simulink model "TopLevelSim"  (R2024b)
settings: Solver=FixedStepDiscrete  StartTime=0.0  StopTime=sysParams.FPGAClkPeriod*1e4  RelTol=1e-3
PreLoadFcn:
  | init;
undefined symbols (not defined in the file): bfCoeffs_fxp, chanConfig, const_16APSK, const_64APSK, FXP, iChain, modEnable, modSel, OFDMmodType, SC, SCmodType, sysParams, tuningWord, txData
libraries: hdlsllib x20, commdigbbndpm3 x8, commdigbbndam3 x8, dspmlti4 x8, dsphdlfiltering2 x8, whdlmod x4, dsphdlsigops2 x4
(part 1 of 2)
settings Model: DataTypeOverride=Off  Creator=aless  LastModifiedBy=aless
settings SolverCC: PositivePriorityOrder=on
settings OptimizationCC: BlockReduction=off  ConditionallyExecuteInputs=off  DefaultParameterBehavior=Inlined  InheritOutputTypeSmallerThanSingle=on  EnhancedBackFolding=on  PassReuseOutputArgsAs=Individual arguments  ZeroExternalMemoryAtStartup=off  ZeroInternalMemoryAtStartup=off  MaxStackSize=64  OptimizeBlockOrder=speed  DifferentSizesBufferReuse=on  OptimizationCustomize=off  EfficientTunableParamExpr=on
settings DebuggingCC: AlgebraicLoopMsg=error  SingleTaskRateTransMsg=warning  ParameterTunabilityLossMsg=error  UnconnectedInputMsg=warning  UnconnectedOutputMsg=warning  UnconnectedLineMsg=warning
settings HardwareCC: ProdBitPerPointer=32  ProdBitPerSizeT=32  ProdBitPerPtrDiffT=32  ProdLargestAtomicFloat=None  ProdIntDivRoundTo=Undefined  ProdEndianess=Unspecified  ProdWordSize=32  ProdHWDeviceType=ASIC/FPGA->ASIC/FPGA  TargetBitPerPointer=64  TargetBitPerSizeT=64  TargetBitPerPtrDiffT=64  TargetLongLongMode=on  TargetIntDivRoundTo=Zero  TargetEndianess=LittleEndian  TargetWordSize=64  TargetHWDeviceType=Custom Processor->MATLAB Host Computer  ProdEqTarget=off  HardwareBoardFeatureSet=SoCBlockset
settings ModelReferenceCC: ModelReferenceNumInstancesAllowed=Single
settings RTWCC: Description=Embedded Coder  SystemTargetFile=ert.tlc  HardwareBoard=Xilinx Zynq UltraScale+ RFSoC ZCU208 Evaluation Kit  TLCOptions="-aInlineSetEventsForThisBaseRateFcn=TLC_FALSE -aSuppressMultiTaskScheduler=TLC_FALSE  -aRateBasedStepFcn=0"  TemplateMakefile=ert_default_tmf  Toolchain=Linaro AArch64 Linux v6.3.1
settings CodeAppCC: ForceParamTrailComments=on  IgnoreCustomStorageClasses=off  OperatorAnnotations=on  SimulinkDataObjDesc=on  SFDataObjDesc=on  InsertBlockDesc=on

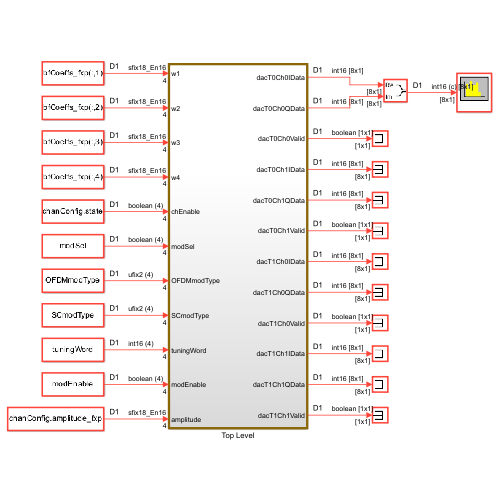
[thumbnail: Simulink's stored preview of the top-level diagram]
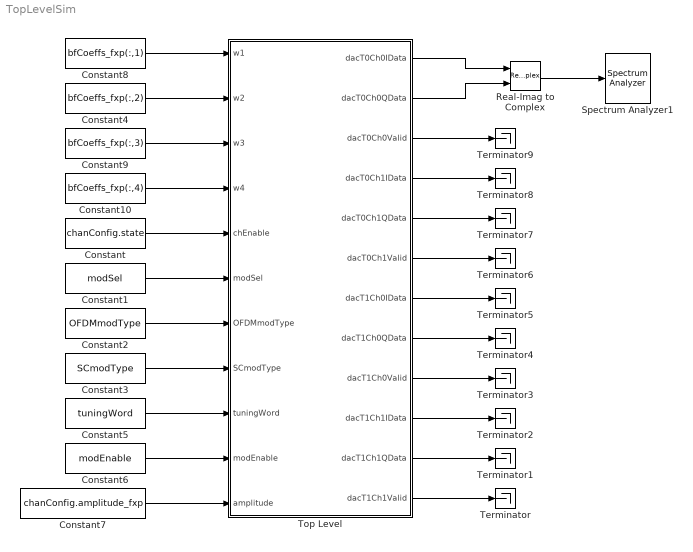
== system TopLevelSim ==
  Constant : Constant  Value=chanConfig.state  OutDataTypeStr=boolean  SampleTime=sysParams.FPGAClkPeriod
  Constant1 : Constant  Value=modSel  OutDataTypeStr=boolean  SampleTime=sysParams.FPGAClkPeriod
  Constant10 : Constant  Value=bfCoeffs_fxp(:,4)  OutDataTypeStr=fixdt(1,FXP.sampWL,FXP.sampFL)  SampleTime=sysParams.FPGAClkPeriod
  Constant2 : Constant  Value=OFDMmodType  OutDataTypeStr=fixdt(0,2,0)  SampleTime=sysParams.FPGAClkPeriod
  Constant3 : Constant  Value=SCmodType  OutDataTypeStr=fixdt(0,2,0)  SampleTime=sysParams.FPGAClkPeriod
  Constant4 : Constant  Value=bfCoeffs_fxp(:,2)  OutDataTypeStr=fixdt(1,FXP.sampWL,FXP.sampFL)  SampleTime=sysParams.FPGAClkPeriod
  Constant5 : Constant  Value=tuningWord  OutDataTypeStr=fixdt(1,FXP.NCOphaseAccWL,0)  SampleTime=sysParams.FPGAClkPeriod
  Constant6 : Constant  Value=modEnable  OutDataTypeStr=boolean  SampleTime=sysParams.FPGAClkPeriod
  Constant7 : Constant  Value=chanConfig.amplitude_fxp  OutDataTypeStr=fixdt(1,FXP.sampWL,FXP.sampFL)  SampleTime=sysParams.FPGAClkPeriod
  Constant8 : Constant  Value=bfCoeffs_fxp(:,1)  OutDataTypeStr=fixdt(1,FXP.sampWL,FXP.sampFL)  SampleTime=sysParams.FPGAClkPeriod
  Constant9 : Constant  Value=bfCoeffs_fxp(:,3)  OutDataTypeStr=fixdt(1,FXP.sampWL,FXP.sampFL)  SampleTime=sysParams.FPGAClkPeriod
  Real-Imag to Complex : RealImagToComplex
  Spectrum Analyzer1 : SpectrumAnalyzer  WindowPosition=[0.000000,36.000000,1536.000000,792.000000,]  ScopeFrameLocation=window  Method=Welch  FrequencyResolutionMethod=Window length  WindowInvariantSamplesPerUpdate=on  WindowLength=4096  FFTLengthSource=Property  FFTLength=8192  Span=1966080000  StartFrequency=-983040000  StopFrequency=983040000  ReferenceLoad=100  YLimits=[-48.29571919,106.76240946]  SelectedToolstripTab=spectrumAnalyzerToolstrip.estimationTab
  Terminator{,1..9} (10 alike) : Terminator
  Top Level : Subsystem  TreatAsAtomicUnit=on
  wires:
  Top Level/1(dacT0Ch0IData) -> Real-Imag to Complex/1
  Top Level/2(dacT0Ch0QData) -> Real-Imag to Complex/2
  Top Level/10(dacT1Ch1IData) -> Terminator2/1
  Top Level/11(dacT1Ch1QData) -> Terminator1/1
  Top Level/12(dacT1Ch1Valid) -> Terminator/1
  Real-Imag to Complex/1 -> Spectrum Analyzer1/1
  Top Level/5(dacT0Ch1QData) -> Terminator7/1
  Top Level/6(dacT0Ch1Valid) -> Terminator6/1
  Top Level/7(dacT1Ch0IData) -> Terminator5/1
  Top Level/8(dacT1Ch0QData) -> Terminator4/1
  Top Level/9(dacT1Ch0Valid) -> Terminator3/1
  Top Level/4(dacT0Ch1IData) -> Terminator8/1
  Top Level/3(dacT0Ch0Valid) -> Terminator9/1
  Constant8/1 -> Top Level/1(w1)
  Constant4/1 -> Top Level/2(w2)
  Constant9/1 -> Top Level/3(w3)
  Constant10/1 -> Top Level/4(w4)
  Constant/1 -> Top Level/5(chEnable)
  Constant1/1 -> Top Level/6(modSel)
  Constant2/1 -> Top Level/7(OFDMmodType)
  Constant3/1 -> Top Level/8(SCmodType)
  Constant5/1 -> Top Level/9(tuningWord)
  Constant6/1 -> Top Level/10(modEnable)
  Constant7/1 -> Top Level/11(amplitude)

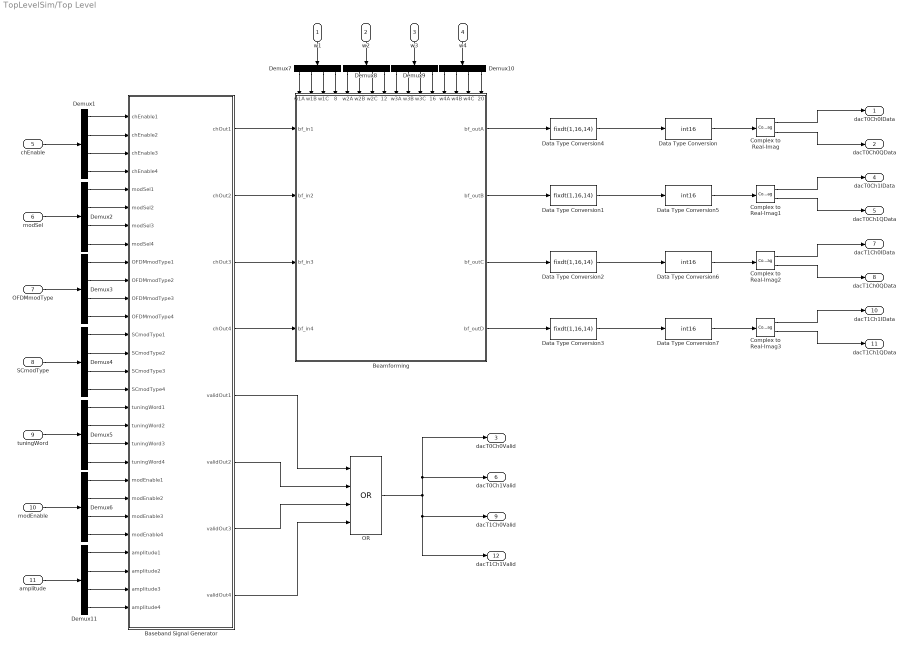
== system TopLevelSim/Top Level ==
  w1 : Inport
  w2 : Inport  Port=2
  w3 : Inport  Port=3
  w4 : Inport  Port=4
  chEnable : Inport  Port=5
  modSel : Inport  Port=6
  OFDMmodType : Inport  Port=7
  SCmodType : Inport  Port=8
  tuningWord : Inport  Port=9
  modEnable : Inport  Port=10
  amplitude : Inport  Port=11
  Baseband Signal Generator : Subsystem
  Beamforming : Subsystem
      settings: PortSchema="{\"entries\":[{\"content\":{\"sides\":[{\"content\":{\"connectorIds\":[\"In1\",\"In2\",\"In3\",\"In4\"]},\"type\":\"ConnectorPlacement.EquallySpacedRectSide\",\"uuid\":\"7b2ca850-5a44-4fe3-a571-bc89de8a8d8a\"},{\"content\":{\"connectorIds\":[\"Out1\",\"Out2\",\"Out3\",\"Out4\"],\"side\":\"RIGHT\"},\"type\":\"ConnectorPlacement.EquallySpacedRectSide\",\"uuid\":\"6a3de6dc-f4ee-4138-b8b6-8ad549f5ffcd\"},{\"content\":{\"connectorIds\":[\"In5\",\"In6\",\"In7\",\"In8\",\"In9\",\"In10\",\"In11\",\"In12\",\"In13\",\"In14\",\"In15\",\"In16\",\"In17\",\"In18\",\"In19\",\"In20\"],\"side\":\"TOP\"},\"type\":\"ConnectorPlacement.EquallySpacedRectSide\",\"uuid\":\"7b227388-a06d-4fee-a646-8c31054e6e12\"}]},\"type\":\"ConnectorPlacement.EquallySpacedConnector\",\"uuid\":\"7849fa84-ba55-4fcd-9e9c-b96e73e847f7\"}],\"packageUris\":[\"http://schema.mathworks.com/mf0/Connector/R2020b\"],\"version\":\"1.0\"}"
  Complex to Real-Imag{,1..3} (4 alike) : ComplexToRealImag
  Data Type Conversion{,5..7} (4 alike) : DataTypeConversion  OutDataTypeStr=int16  ConvertRealWorld=Stored Integer (SI)  SaturateOnIntegerOverflow=off  RndMeth=Floor  LockScale=on
  Data Type Conversion{1..4} (4 alike) : DataTypeConversion  OutDataTypeStr=fixdt(1,16,14)  RndMeth=Nearest  SaturateOnIntegerOverflow=off
  Demux{1..11} (11 alike) : Demux
  OR : Logic  Operator=OR  Inputs=4  AllPortsSameDT=off  OutDataTypeStr=boolean
  dacT0Ch0IData : Outport
  dacT0Ch0QData : Outport  Port=2
  dacT0Ch0Valid : Outport  Port=3
  dacT0Ch1IData : Outport  Port=4
  dacT0Ch1QData : Outport  Port=5
  dacT0Ch1Valid : Outport  Port=6
  dacT1Ch0IData : Outport  Port=7
  dacT1Ch0QData : Outport  Port=8
  dacT1Ch0Valid : Outport  Port=9
  dacT1Ch1IData : Outport  Port=10
  dacT1Ch1QData : Outport  Port=11
  dacT1Ch1Valid : Outport  Port=12
  wires:
  chEnable/1 -> Demux1/1
  SCmodType/1 -> Demux4/1
  OFDMmodType/1 -> Demux3/1
  modSel/1 -> Demux2/1
  modEnable/1 -> Demux6/1
  Data Type Conversion3/1 -> Data Type Conversion7/1
  Complex to Real-Imag3/2 -> dacT1Ch1QData/1
  Baseband Signal Generator/7(validOut3) -> OR/3
  Baseband Signal Generator/3(chOut3) -> Beamforming/3(bf_in3)
  Complex to Real-Imag2/2 -> dacT1Ch0QData/1
  Complex to Real-Imag1/2 -> dacT0Ch1QData/1
  Data Type Conversion2/1 -> Data Type Conversion6/1
  Complex to Real-Imag/1 -> dacT0Ch0IData/1
  Data Type Conversion7/1 -> Complex to Real-Imag3/1
  OR/1 -> dacT0Ch0Valid/1, dacT0Ch1Valid/1, dacT1Ch1Valid/1, dacT1Ch0Valid/1
  Demux7/1 -> Beamforming/5(w1A)
  Beamforming/1(bf_outA) -> Data Type Conversion4/1
  Baseband Signal Generator/6(validOut2) -> OR/2
  Baseband Signal Generator/5(validOut1) -> OR/1
  Complex to Real-Imag1/1 -> dacT0Ch1IData/1
  Complex to Real-Imag2/1 -> dacT1Ch0IData/1
  Baseband Signal Generator/8(validOut4) -> OR/4
  Complex to Real-Imag/2 -> dacT0Ch0QData/1
  Data Type Conversion4/1 -> Data Type Conversion/1
  Baseband Signal Generator/4(chOut4) -> Beamforming/4(bf_in4)
  Baseband Signal Generator/1(chOut1) -> Beamforming/1(bf_in1)
  Beamforming/2(bf_outB) -> Data Type Conversion1/1
  Complex to Real-Imag3/1 -> dacT1Ch1IData/1
  Data Type Conversion6/1 -> Complex to Real-Imag2/1
  Beamforming/4(bf_outD) -> Data Type Conversion3/1
  Data Type Conversion5/1 -> Complex to Real-Imag1/1
  Data Type Conversion1/1 -> Data Type Conversion5/1
  Beamforming/3(bf_outC) -> Data Type Conversion2/1
  Data Type Conversion/1 -> Complex to Real-Imag/1
  Baseband Signal Generator/2(chOut2) -> Beamforming/2(bf_in2)
  Demux7/2 -> Beamforming/6(w1B)
  Demux7/3 -> Beamforming/7(w1C)
  Demux7/4 -> Beamforming/8(w1D)
  Demux8/2 -> Beamforming/10(w2B)
  Demux8/3 -> Beamforming/11(w2C)
  Demux8/4 -> Beamforming/12(w2D)
  Demux8/1 -> Beamforming/9(w2A)
  Demux9/2 -> Beamforming/14(w3B)
  Demux9/3 -> Beamforming/15(w3C)
  Demux9/4 -> Beamforming/16(w3D)
  Demux9/1 -> Beamforming/13(w3A)
  Demux10/2 -> Beamforming/18(w4B)
  Demux10/3 -> Beamforming/19(w4C)
  Demux10/4 -> Beamforming/20(w4D)
  Demux10/1 -> Beamforming/17(w4A)
  w1/1 -> Demux7/1
  w2/1 -> Demux8/1
  w3/1 -> Demux9/1
  w4/1 -> Demux10/1
  tuningWord/1 -> Demux5/1
  amplitude/1 -> Demux11/1
  Demux1/1 -> Baseband Signal Generator/1(chEnable1)
  Demux1/2 -> Baseband Signal Generator/2(chEnable2)
  Demux1/3 -> Baseband Signal Generator/3(chEnable3)
  Demux1/4 -> Baseband Signal Generator/4(chEnable4)
  Demux2/1 -> Baseband Signal Generator/5(modSel1)
  Demux2/2 -> Baseband Signal Generator/6(modSel2)
  Demux2/3 -> Baseband Signal Generator/7(modSel3)
  Demux2/4 -> Baseband Signal Generator/8(modSel4)
  Demux3/1 -> Baseband Signal Generator/9(OFDMmodType1)
  Demux3/2 -> Baseband Signal Generator/10(OFDMmodType2)
  Demux3/3 -> Baseband Signal Generator/11(OFDMmodType3)
  Demux3/4 -> Baseband Signal Generator/12(OFDMmodType4)
  Demux4/1 -> Baseband Signal Generator/13(SCmodType1)
  Demux4/2 -> Baseband Signal Generator/14(SCmodType2)
  Demux4/3 -> Baseband Signal Generator/15(SCmodType3)
  Demux4/4 -> Baseband Signal Generator/16(SCmodType4)
  Demux5/1 -> Baseband Signal Generator/17(tuningWord1)
  Demux5/2 -> Baseband Signal Generator/18(tuningWord2)
  Demux5/3 -> Baseband Signal Generator/19(tuningWord3)
  Demux5/4 -> Baseband Signal Generator/20(tuningWord4)
  Demux6/1 -> Baseband Signal Generator/21(modEnable1)
  Demux6/2 -> Baseband Signal Generator/22(modEnable2)
  Demux6/3 -> Baseband Signal Generator/23(modEnable3)
  Demux6/4 -> Baseband Signal Generator/24(modEnable4)
  Demux11/1 -> Baseband Signal Generator/25(amplitude1)
  Demux11/2 -> Baseband Signal Generator/26(amplitude2)
  Demux11/3 -> Baseband Signal Generator/27(amplitude3)
  Demux11/4 -> Baseband Signal Generator/28(amplitude4)

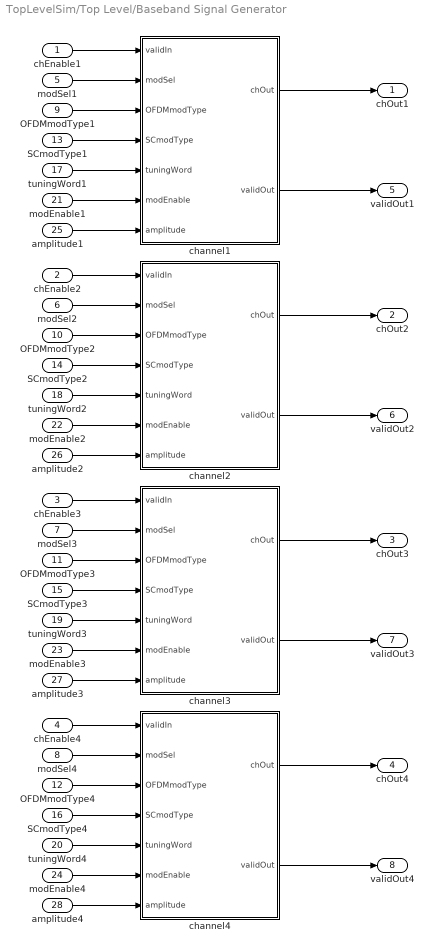
== system TopLevelSim/Top Level/Baseband Signal Generator ==
  chEnable1 : Inport
  chEnable2 : Inport  Port=2
  chEnable3 : Inport  Port=3
  chEnable4 : Inport  Port=4
  modSel1 : Inport  Port=5
  modSel2 : Inport  Port=6
  modSel3 : Inport  Port=7
  modSel4 : Inport  Port=8
  OFDMmodType1 : Inport  Port=9
  OFDMmodType2 : Inport  Port=10
  OFDMmodType3 : Inport  Port=11
  OFDMmodType4 : Inport  Port=12
  SCmodType1 : Inport  Port=13
  SCmodType2 : Inport  Port=14
  SCmodType3 : Inport  Port=15
  SCmodType4 : Inport  Port=16
  tuningWord1 : Inport  Port=17
  tuningWord2 : Inport  Port=18
  tuningWord3 : Inport  Port=19
  tuningWord4 : Inport  Port=20
  modEnable1 : Inport  Port=21
  modEnable2 : Inport  Port=22
  modEnable3 : Inport  Port=23
  modEnable4 : Inport  Port=24
  amplitude1 : Inport  Port=25
  amplitude2 : Inport  Port=26
  amplitude3 : Inport  Port=27
  amplitude4 : Inport  Port=28
  channel1 : Subsystem
  channel2 : Subsystem
  channel3 : Subsystem
  channel4 : Subsystem
  chOut1 : Outport
  chOut2 : Outport  Port=2
  chOut3 : Outport  Port=3
  chOut4 : Outport  Port=4
  validOut1 : Outport  Port=5
  validOut2 : Outport  Port=6
  validOut3 : Outport  Port=7
  validOut4 : Outport  Port=8
  wires:
  tuningWord4/1 -> channel4/5(tuningWord)
  modEnable4/1 -> channel4/6(modEnable)
  modEnable2/1 -> channel2/6(modEnable)
  modEnable1/1 -> channel1/6(modEnable)
  OFDMmodType1/1 -> channel1/3(OFDMmodType)
  modSel1/1 -> channel1/2(modSel)
  tuningWord1/1 -> channel1/5(tuningWord)
  OFDMmodType3/1 -> channel3/3(OFDMmodType)
  channel3/2(validOut) -> validOut3/1
  channel2/1(chOut) -> chOut2/1
  SCmodType1/1 -> channel1/4(SCmodType)
  chEnable2/1 -> channel2/1(validIn)
  channel4/1(chOut) -> chOut4/1
  chEnable1/1 -> channel1/1(validIn)
  channel2/2(validOut) -> validOut2/1
  amplitude1/1 -> channel1/7(amplitude)
  SCmodType3/1 -> channel3/4(SCmodType)
  amplitude4/1 -> channel4/7(amplitude)
  SCmodType4/1 -> channel4/4(SCmodType)
  chEnable4/1 -> channel4/1(validIn)
  modSel4/1 -> channel4/2(modSel)
  OFDMmodType4/1 -> channel4/3(OFDMmodType)
  amplitude2/1 -> channel2/7(amplitude)
  OFDMmodType2/1 -> channel2/3(OFDMmodType)
  SCmodType2/1 -> channel2/4(SCmodType)
  tuningWord3/1 -> channel3/5(tuningWord)
  modSel2/1 -> channel2/2(modSel)
  tuningWord2/1 -> channel2/5(tuningWord)
  modEnable3/1 -> channel3/6(modEnable)
  modSel3/1 -> channel3/2(modSel)
  amplitude3/1 -> channel3/7(amplitude)
  chEnable3/1 -> channel3/1(validIn)
  channel3/1(chOut) -> chOut3/1
  channel4/2(validOut) -> validOut4/1
  channel1/1(chOut) -> chOut1/1
  channel1/2(validOut) -> validOut1/1

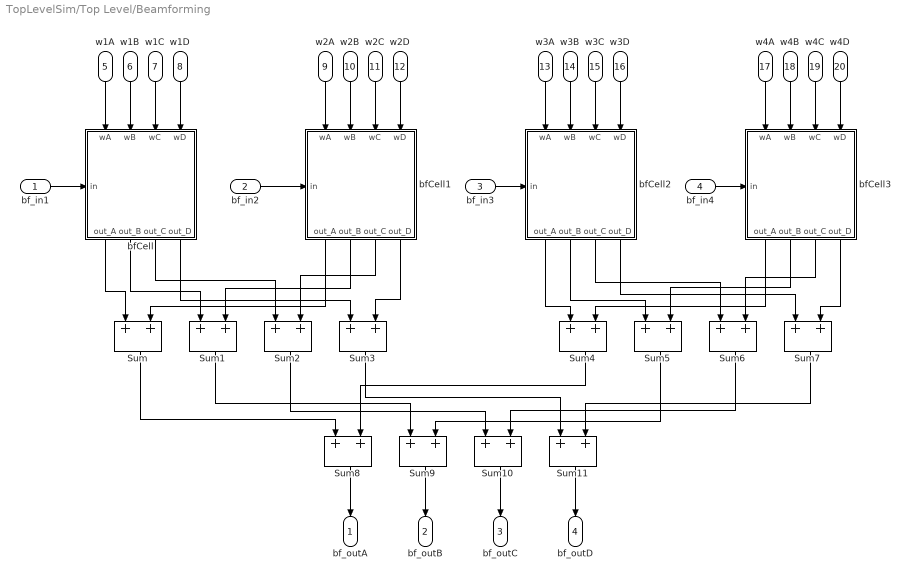
== system TopLevelSim/Top Level/Beamforming ==
  bf_in1 : Inport
  bf_in2 : Inport  Port=2
  bf_in3 : Inport  Port=3
  bf_in4 : Inport  Port=4
  w1A : Inport  Port=5
  w1B : Inport  Port=6
  w1C : Inport  Port=7
  w1D : Inport  Port=8
  w2A : Inport  Port=9
  w2B : Inport  Port=10
  w2C : Inport  Port=11
  w2D : Inport  Port=12
  w3A : Inport  Port=13
  w3B : Inport  Port=14
  w3C : Inport  Port=15
  w3D : Inport  Port=16
  w4A : Inport  Port=17
  w4B : Inport  Port=18
  w4C : Inport  Port=19
  w4D : Inport  Port=20
  Sum{,1..11} (12 alike) : Sum  OutDataTypeStr=Inherit: Same as first input
  bfCell : Subsystem
      settings: PortSchema="{\"entries\":[{\"content\":{\"sides\":[{\"content\":{\"connectorIds\":[\"In1\",\"In2\",\"In3\",\"In4\"]},\"type\":\"ConnectorPlacement.EquallySpacedRectSide\",\"uuid\":\"0c826d6a-73c9-4dba-b1c5-31cfcef02303\"},{\"content\":{\"connectorIds\":[\"Out1\",\"Out2\",\"Out3\",\"Out4\"],\"side\":\"RIGHT\"},\"type\":\"ConnectorPlacement.EquallySpacedRectSide\",\"uuid\":\"e2d5e3de-4ff0-416d-bc8f-a95d356a0a64\"},{\"content\":{\"connectorIds\":[\"In5\"],\"side\":\"TOP\"},\"type\":\"ConnectorPlacement.EquallySpacedRectSide\",\"uuid\":\"bc2266f3-9c70-485a-9b9f-6558f87275cb\"}]},\"type\":\"ConnectorPlacement.EquallySpacedConnector\",\"uuid\":\"4675a578-71f2-44f5-ac97-67035b521010\"}],\"packageUris\":[\"http://schema.mathworks.com/mf0/Connector/R2020b\"],\"version\":\"1.0\"}"
  bfCell1 : Subsystem
      settings: PortSchema="{\"entries\":[{\"content\":{\"sides\":[{\"content\":{\"connectorIds\":[\"In1\",\"In2\",\"In3\",\"In4\"]},\"type\":\"ConnectorPlacement.EquallySpacedRectSide\",\"uuid\":\"0c826d6a-73c9-4dba-b1c5-31cfcef02303\"},{\"content\":{\"connectorIds\":[\"Out1\",\"Out2\",\"Out3\",\"Out4\"],\"side\":\"RIGHT\"},\"type\":\"ConnectorPlacement.EquallySpacedRectSide\",\"uuid\":\"e2d5e3de-4ff0-416d-bc8f-a95d356a0a64\"},{\"content\":{\"connectorIds\":[\"In5\"],\"side\":\"TOP\"},\"type\":\"ConnectorPlacement.EquallySpacedRectSide\",\"uuid\":\"bc2266f3-9c70-485a-9b9f-6558f87275cb\"}]},\"type\":\"ConnectorPlacement.EquallySpacedConnector\",\"uuid\":\"4675a578-71f2-44f5-ac97-67035b521010\"}],\"packageUris\":[\"http://schema.mathworks.com/mf0/Connector/R2020b\"],\"version\":\"1.0\"}"
  bfCell2 : Subsystem
      settings: PortSchema="{\"entries\":[{\"content\":{\"sides\":[{\"content\":{\"connectorIds\":[\"In1\",\"In2\",\"In3\",\"In4\"]},\"type\":\"ConnectorPlacement.EquallySpacedRectSide\",\"uuid\":\"0c826d6a-73c9-4dba-b1c5-31cfcef02303\"},{\"content\":{\"connectorIds\":[\"Out1\",\"Out2\",\"Out3\",\"Out4\"],\"side\":\"RIGHT\"},\"type\":\"ConnectorPlacement.EquallySpacedRectSide\",\"uuid\":\"e2d5e3de-4ff0-416d-bc8f-a95d356a0a64\"},{\"content\":{\"connectorIds\":[\"In5\"],\"side\":\"TOP\"},\"type\":\"ConnectorPlacement.EquallySpacedRectSide\",\"uuid\":\"bc2266f3-9c70-485a-9b9f-6558f87275cb\"}]},\"type\":\"ConnectorPlacement.EquallySpacedConnector\",\"uuid\":\"4675a578-71f2-44f5-ac97-67035b521010\"}],\"packageUris\":[\"http://schema.mathworks.com/mf0/Connector/R2020b\"],\"version\":\"1.0\"}"
  bfCell3 : Subsystem
      settings: PortSchema="{\"entries\":[{\"content\":{\"sides\":[{\"content\":{\"connectorIds\":[\"In1\",\"In2\",\"In3\",\"In4\"]},\"type\":\"ConnectorPlacement.EquallySpacedRectSide\",\"uuid\":\"0c826d6a-73c9-4dba-b1c5-31cfcef02303\"},{\"content\":{\"connectorIds\":[\"Out1\",\"Out2\",\"Out3\",\"Out4\"],\"side\":\"RIGHT\"},\"type\":\"ConnectorPlacement.EquallySpacedRectSide\",\"uuid\":\"e2d5e3de-4ff0-416d-bc8f-a95d356a0a64\"},{\"content\":{\"connectorIds\":[\"In5\"],\"side\":\"TOP\"},\"type\":\"ConnectorPlacement.EquallySpacedRectSide\",\"uuid\":\"bc2266f3-9c70-485a-9b9f-6558f87275cb\"}]},\"type\":\"ConnectorPlacement.EquallySpacedConnector\",\"uuid\":\"4675a578-71f2-44f5-ac97-67035b521010\"}],\"packageUris\":[\"http://schema.mathworks.com/mf0/Connector/R2020b\"],\"version\":\"1.0\"}"
  bf_outA : Outport
  bf_outB : Outport  Port=2
  bf_outC : Outport  Port=3
  bf_outD : Outport  Port=4
  wires:
  Sum8/1 -> bf_outA/1
  Sum9/1 -> bf_outB/1
  Sum10/1 -> bf_outC/1
  Sum11/1 -> bf_outD/1
  w1B/1 -> bfCell/2(wB)
  w1D/1 -> bfCell/4(wD)
  w1A/1 -> bfCell/1(wA)
  w1C/1 -> bfCell/3(wC)
  w2A/1 -> bfCell1/1(wA)
  w2B/1 -> bfCell1/2(wB)
  w2C/1 -> bfCell1/3(wC)
  w2D/1 -> bfCell1/4(wD)
  w3A/1 -> bfCell2/1(wA)
  w3B/1 -> bfCell2/2(wB)
  w3C/1 -> bfCell2/3(wC)
  w3D/1 -> bfCell2/4(wD)
  w4A/1 -> bfCell3/1(wA)
  w4B/1 -> bfCell3/2(wB)
  w4C/1 -> bfCell3/3(wC)
  w4D/1 -> bfCell3/4(wD)
  bf_in1/1 -> bfCell/5(in)
  bf_in2/1 -> bfCell1/5(in)
  bf_in3/1 -> bfCell2/5(in)
  bf_in4/1 -> bfCell3/5(in)
  bfCell/1(out_A) -> Sum/1
  bfCell1/1(out_A) -> Sum/2
  bfCell/2(out_B) -> Sum1/1
  bfCell1/2(out_B) -> Sum1/2
  bfCell/3(out_C) -> Sum2/1
  bfCell1/3(out_C) -> Sum2/2
  bfCell/4(out_D) -> Sum3/1
  bfCell1/4(out_D) -> Sum3/2
  bfCell2/1(out_A) -> Sum4/1
  bfCell3/1(out_A) -> Sum4/2
  bfCell2/2(out_B) -> Sum5/1
  bfCell3/2(out_B) -> Sum5/2
  bfCell2/3(out_C) -> Sum6/1
  bfCell3/3(out_C) -> Sum6/2
  bfCell2/4(out_D) -> Sum7/1
  bfCell3/4(out_D) -> Sum7/2
  Sum/1 -> Sum8/1
  Sum4/1 -> Sum8/2
  Sum1/1 -> Sum9/1
  Sum2/1 -> Sum10/1
  Sum5/1 -> Sum9/2
  Sum6/1 -> Sum10/2
  Sum3/1 -> Sum11/1
  Sum7/1 -> Sum11/2

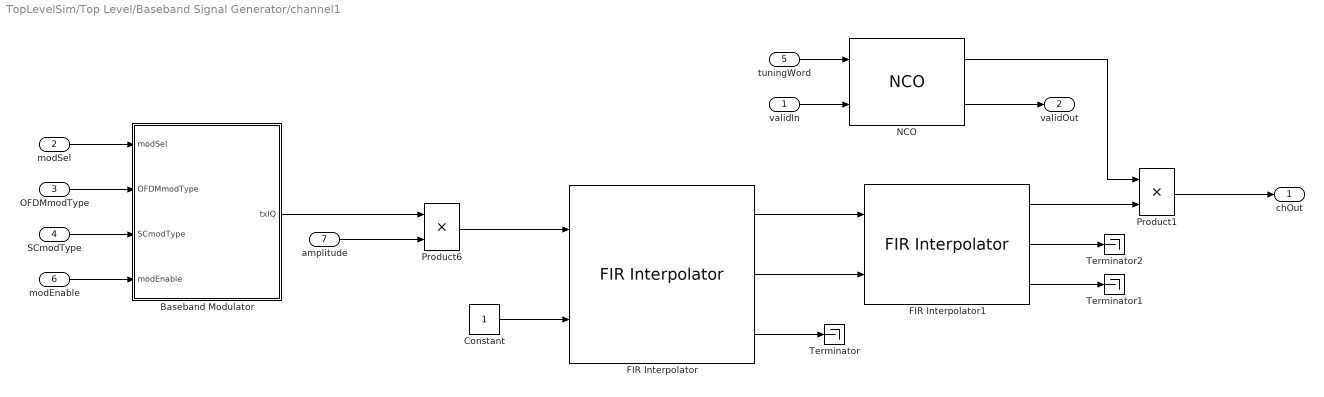
== system TopLevelSim/Top Level/Baseband Signal Generator/channel1 ==
  validIn : Inport
  modSel : Inport  Port=2
  OFDMmodType : Inport  Port=3
  SCmodType : Inport  Port=4
  tuningWord : Inport  Port=5
  modEnable : Inport  Port=6
  amplitude : Inport  Port=7
  Baseband Modulator : Subsystem
  Constant : Constant  OutDataTypeStr=boolean  SampleTime=sysParams.FPGAClkPeriod
  FIR Interpolator : dsphdlfiltering2/FIR Interpolator  Numerator=iChain.firTaps  FilterStructure=Direct form systolic  InterpolationFactor=4  NumCycles=1  OptimizeSymmCoeff=on  SimulateUsing=Code generation  roundingMode=Floor  overflowMode=off  CoefficientsDataTypeStr=fixdt(1,FXP.coeffWL,FXP.coeffFL)  OutputDataTypeStr=fixdt(1,FXP.sampWL,FXP.sampFL)  ResetInputPort=off  HDLGlobalReset=off
  FIR Interpolator1 : dsphdlfiltering2/FIR Interpolator  Numerator=iChain.hbTaps  FilterStructure=Direct form systolic  InterpolationFactor=2  NumCycles=1  OptimizeSymmCoeff=off  SimulateUsing=Code generation  roundingMode=Floor  overflowMode=off  CoefficientsDataTypeStr=fixdt(1,FXP.coeffWL,FXP.coeffFL)  OutputDataTypeStr=fixdt(1,FXP.sampWL,FXP.sampFL)  ResetInputPort=off  HDLGlobalReset=off
  NCO : dsphdlsigops2/NCO  PhaseIncrementSource=Input port  PhaseIncrement=100  PhaseOffsetSource=Property  PhaseOffset=0  DitherSource=None  NumDitherBits=4  SamplesPerFrame=iChain.interpFactor  LUTCompress=on  ResetAction=off  Waveform=Complex exponential  PhasePort=off  SimulateUsing=Code generation  AccumulatorWL=FXP.NCOphaseAccWL  PhaseQuantization=on  NumQuantizerAccumulatorBits=FXP.NCOlutAddressWL  OutputDataType=Binary point scaling  OutputWL=FXP.sampWL  OutputFL=FXP.sampFL
  Product1 : Product  OutDataTypeStr=fixdt(1,FXP.sampWL,FXP.sampFL)
  Product6 : Product  OutDataTypeStr=fixdt(1,FXP.sampWL,FXP.sampFL)
  Terminator : Terminator
  Terminator1 : Terminator
  Terminator2 : Terminator
  chOut : Outport
  validOut : Outport  Port=2
  wires:
  FIR Interpolator1/3 -> Terminator1/1
  SCmodType/1 -> Baseband Modulator/3(SCmodType)
  tuningWord/1 -> NCO/1
  modSel/1 -> Baseband Modulator/1(modSel)
  OFDMmodType/1 -> Baseband Modulator/2(OFDMmodType)
  modEnable/1 -> Baseband Modulator/4(modEnable)
  FIR Interpolator/3 -> Terminator/1
  Baseband Modulator/1(txIQ) -> Product6/1
  validIn/1 -> NCO/2
  amplitude/1 -> Product6/2
  Product6/1 -> FIR Interpolator/1
  Product1/1 -> chOut/1
  FIR Interpolator/1 -> FIR Interpolator1/1
  FIR Interpolator/2 -> FIR Interpolator1/2
  NCO/2 -> validOut/1
  Constant/1 -> FIR Interpolator/2
  FIR Interpolator1/2 -> Terminator2/1
  FIR Interpolator1/1 -> Product1/2
  NCO/1 -> Product1/1

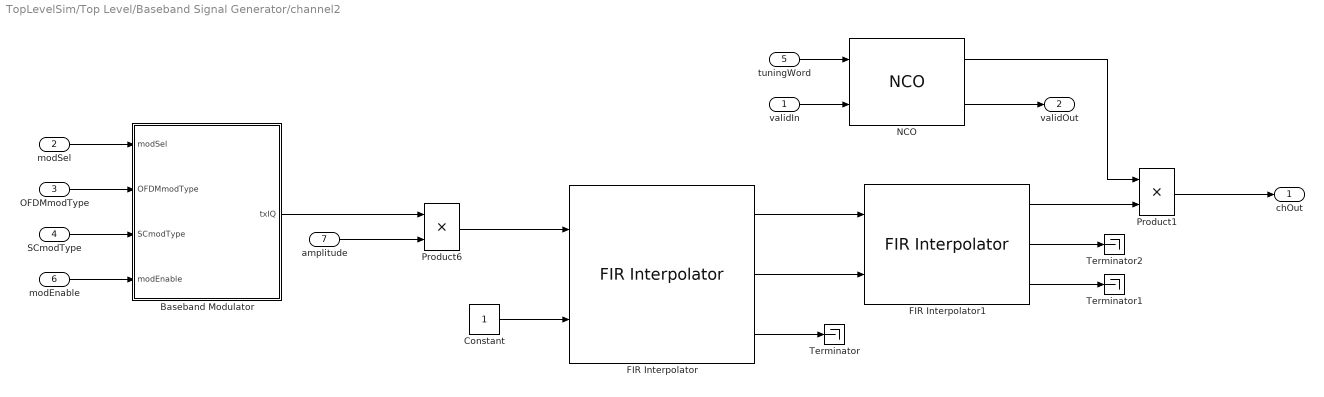
== system TopLevelSim/Top Level/Baseband Signal Generator/channel2 ==
  validIn : Inport
  modSel : Inport  Port=2
  OFDMmodType : Inport  Port=3
  SCmodType : Inport  Port=4
  tuningWord : Inport  Port=5
  modEnable : Inport  Port=6
  amplitude : Inport  Port=7
  Baseband Modulator : Subsystem
  Constant : Constant  OutDataTypeStr=boolean  SampleTime=sysParams.FPGAClkPeriod
  FIR Interpolator : dsphdlfiltering2/FIR Interpolator  Numerator=iChain.firTaps  FilterStructure=Direct form systolic  InterpolationFactor=4  NumCycles=1  OptimizeSymmCoeff=on  SimulateUsing=Code generation  roundingMode=Floor  overflowMode=off  CoefficientsDataTypeStr=fixdt(1,FXP.coeffWL,FXP.coeffFL)  OutputDataTypeStr=fixdt(1,FXP.sampWL,FXP.sampFL)  ResetInputPort=off  HDLGlobalReset=off
  FIR Interpolator1 : dsphdlfiltering2/FIR Interpolator  Numerator=iChain.hbTaps  FilterStructure=Direct form systolic  InterpolationFactor=2  NumCycles=1  OptimizeSymmCoeff=off  SimulateUsing=Code generation  roundingMode=Floor  overflowMode=off  CoefficientsDataTypeStr=fixdt(1,FXP.coeffWL,FXP.coeffFL)  OutputDataTypeStr=fixdt(1,FXP.sampWL,FXP.sampFL)  ResetInputPort=off  HDLGlobalReset=off
  NCO : dsphdlsigops2/NCO  PhaseIncrementSource=Input port  PhaseIncrement=100  PhaseOffsetSource=Property  PhaseOffset=0  DitherSource=None  NumDitherBits=4  SamplesPerFrame=iChain.interpFactor  LUTCompress=on  ResetAction=off  Waveform=Complex exponential  PhasePort=off  SimulateUsing=Code generation  AccumulatorWL=FXP.NCOphaseAccWL  PhaseQuantization=on  NumQuantizerAccumulatorBits=FXP.NCOlutAddressWL  OutputDataType=Binary point scaling  OutputWL=FXP.sampWL  OutputFL=FXP.sampFL
  Product1 : Product  OutDataTypeStr=fixdt(1,FXP.sampWL,FXP.sampFL)
  Product6 : Product  OutDataTypeStr=fixdt(1,FXP.sampWL,FXP.sampFL)
  Terminator : Terminator
  Terminator1 : Terminator
  Terminator2 : Terminator
  chOut : Outport
  validOut : Outport  Port=2
  wires:
  NCO/1 -> Product1/1
  FIR Interpolator1/1 -> Product1/2
  FIR Interpolator1/2 -> Terminator2/1
  Constant/1 -> FIR Interpolator/2
  NCO/2 -> validOut/1
  FIR Interpolator/2 -> FIR Interpolator1/2
  FIR Interpolator/1 -> FIR Interpolator1/1
  Product1/1 -> chOut/1
  Product6/1 -> FIR Interpolator/1
  amplitude/1 -> Product6/2
  validIn/1 -> NCO/2
  Baseband Modulator/1(txIQ) -> Product6/1
  FIR Interpolator/3 -> Terminator/1
  modEnable/1 -> Baseband Modulator/4(modEnable)
  OFDMmodType/1 -> Baseband Modulator/2(OFDMmodType)
  modSel/1 -> Baseband Modulator/1(modSel)
  tuningWord/1 -> NCO/1
  SCmodType/1 -> Baseband Modulator/3(SCmodType)
  FIR Interpolator1/3 -> Terminator1/1

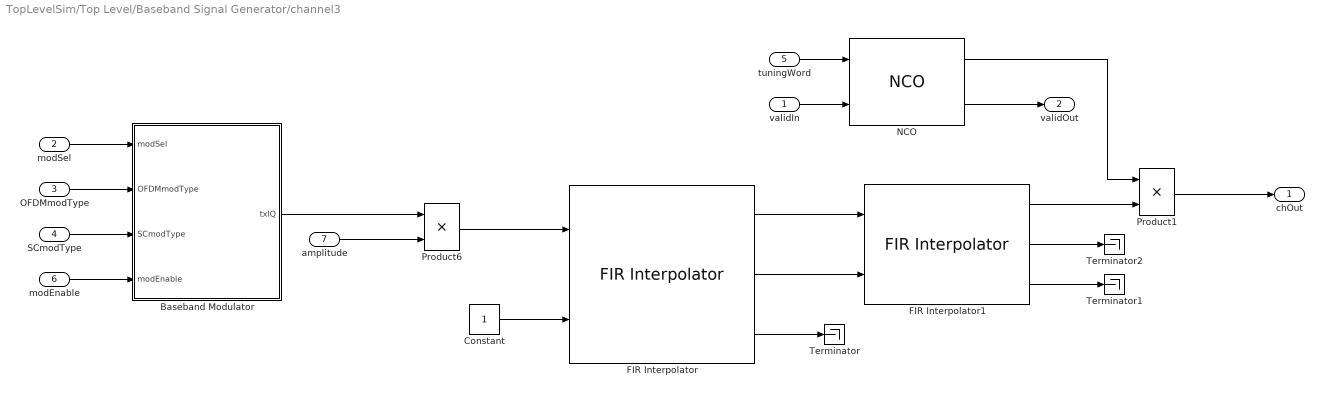
== system TopLevelSim/Top Level/Baseband Signal Generator/channel3 ==
  validIn : Inport
  modSel : Inport  Port=2
  OFDMmodType : Inport  Port=3
  SCmodType : Inport  Port=4
  tuningWord : Inport  Port=5
  modEnable : Inport  Port=6
  amplitude : Inport  Port=7
  Baseband Modulator : Subsystem
  Constant : Constant  OutDataTypeStr=boolean  SampleTime=sysParams.FPGAClkPeriod
  FIR Interpolator : dsphdlfiltering2/FIR Interpolator  Numerator=iChain.firTaps  FilterStructure=Direct form systolic  InterpolationFactor=4  NumCycles=1  OptimizeSymmCoeff=on  SimulateUsing=Code generation  roundingMode=Floor  overflowMode=off  CoefficientsDataTypeStr=fixdt(1,FXP.coeffWL,FXP.coeffFL)  OutputDataTypeStr=fixdt(1,FXP.sampWL,FXP.sampFL)  ResetInputPort=off  HDLGlobalReset=off
  FIR Interpolator1 : dsphdlfiltering2/FIR Interpolator  Numerator=iChain.hbTaps  FilterStructure=Direct form systolic  InterpolationFactor=2  NumCycles=1  OptimizeSymmCoeff=off  SimulateUsing=Code generation  roundingMode=Floor  overflowMode=off  CoefficientsDataTypeStr=fixdt(1,FXP.coeffWL,FXP.coeffFL)  OutputDataTypeStr=fixdt(1,FXP.sampWL,FXP.sampFL)  ResetInputPort=off  HDLGlobalReset=off
  NCO : dsphdlsigops2/NCO  PhaseIncrementSource=Input port  PhaseIncrement=100  PhaseOffsetSource=Property  PhaseOffset=0  DitherSource=None  NumDitherBits=4  SamplesPerFrame=iChain.interpFactor  LUTCompress=on  ResetAction=off  Waveform=Complex exponential  PhasePort=off  SimulateUsing=Code generation  AccumulatorWL=FXP.NCOphaseAccWL  PhaseQuantization=on  NumQuantizerAccumulatorBits=FXP.NCOlutAddressWL  OutputDataType=Binary point scaling  OutputWL=FXP.sampWL  OutputFL=FXP.sampFL
  Product1 : Product  OutDataTypeStr=fixdt(1,FXP.sampWL,FXP.sampFL)
  Product6 : Product  OutDataTypeStr=fixdt(1,FXP.sampWL,FXP.sampFL)
  Terminator : Terminator
  Terminator1 : Terminator
  Terminator2 : Terminator
  chOut : Outport
  validOut : Outport  Port=2
  wires:
  FIR Interpolator1/3 -> Terminator1/1
  SCmodType/1 -> Baseband Modulator/3(SCmodType)
  tuningWord/1 -> NCO/1
  modSel/1 -> Baseband Modulator/1(modSel)
  OFDMmodType/1 -> Baseband Modulator/2(OFDMmodType)
  modEnable/1 -> Baseband Modulator/4(modEnable)
  FIR Interpolator/3 -> Terminator/1
  Baseband Modulator/1(txIQ) -> Product6/1
  validIn/1 -> NCO/2
  amplitude/1 -> Product6/2
  Product6/1 -> FIR Interpolator/1
  Product1/1 -> chOut/1
  FIR Interpolator/1 -> FIR Interpolator1/1
  FIR Interpolator/2 -> FIR Interpolator1/2
  NCO/2 -> validOut/1
  Constant/1 -> FIR Interpolator/2
  FIR Interpolator1/2 -> Terminator2/1
  FIR Interpolator1/1 -> Product1/2
  NCO/1 -> Product1/1

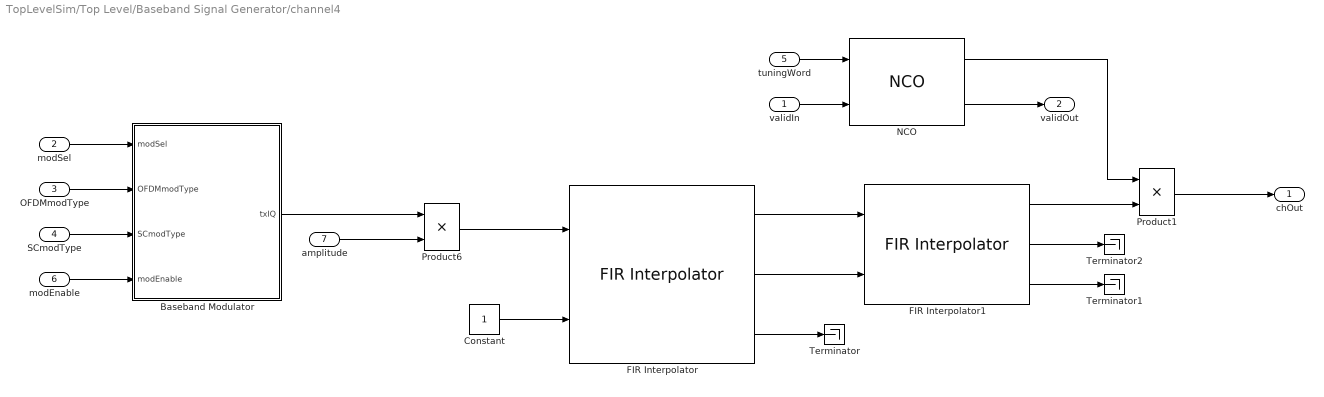
== system TopLevelSim/Top Level/Baseband Signal Generator/channel4 ==
  validIn : Inport
  modSel : Inport  Port=2
  OFDMmodType : Inport  Port=3
  SCmodType : Inport  Port=4
  tuningWord : Inport  Port=5
  modEnable : Inport  Port=6
  amplitude : Inport  Port=7
  Baseband Modulator : Subsystem
  Constant : Constant  OutDataTypeStr=boolean  SampleTime=sysParams.FPGAClkPeriod
  FIR Interpolator : dsphdlfiltering2/FIR Interpolator  Numerator=iChain.firTaps  FilterStructure=Direct form systolic  InterpolationFactor=4  NumCycles=1  OptimizeSymmCoeff=on  SimulateUsing=Code generation  roundingMode=Floor  overflowMode=off  CoefficientsDataTypeStr=fixdt(1,FXP.coeffWL,FXP.coeffFL)  OutputDataTypeStr=fixdt(1,FXP.sampWL,FXP.sampFL)  ResetInputPort=off  HDLGlobalReset=off
  FIR Interpolator1 : dsphdlfiltering2/FIR Interpolator  Numerator=iChain.hbTaps  FilterStructure=Direct form systolic  InterpolationFactor=2  NumCycles=1  OptimizeSymmCoeff=off  SimulateUsing=Code generation  roundingMode=Floor  overflowMode=off  CoefficientsDataTypeStr=fixdt(1,FXP.coeffWL,FXP.coeffFL)  OutputDataTypeStr=fixdt(1,FXP.sampWL,FXP.sampFL)  ResetInputPort=off  HDLGlobalReset=off
  NCO : dsphdlsigops2/NCO  PhaseIncrementSource=Input port  PhaseIncrement=100  PhaseOffsetSource=Property  PhaseOffset=0  DitherSource=None  NumDitherBits=4  SamplesPerFrame=iChain.interpFactor  LUTCompress=on  ResetAction=off  Waveform=Complex exponential  PhasePort=off  SimulateUsing=Code generation  AccumulatorWL=FXP.NCOphaseAccWL  PhaseQuantization=on  NumQuantizerAccumulatorBits=FXP.NCOlutAddressWL  OutputDataType=Binary point scaling  OutputWL=FXP.sampWL  OutputFL=FXP.sampFL
  Product1 : Product  OutDataTypeStr=fixdt(1,FXP.sampWL,FXP.sampFL)
  Product6 : Product  OutDataTypeStr=fixdt(1,FXP.sampWL,FXP.sampFL)
  Terminator : Terminator
  Terminator1 : Terminator
  Terminator2 : Terminator
  chOut : Outport
  validOut : Outport  Port=2
  wires:
  NCO/1 -> Product1/1
  FIR Interpolator1/1 -> Product1/2
  FIR Interpolator1/2 -> Terminator2/1
  Constant/1 -> FIR Interpolator/2
  NCO/2 -> validOut/1
  FIR Interpolator/2 -> FIR Interpolator1/2
  FIR Interpolator/1 -> FIR Interpolator1/1
  Product1/1 -> chOut/1
  Product6/1 -> FIR Interpolator/1
  amplitude/1 -> Product6/2
  validIn/1 -> NCO/2
  Baseband Modulator/1(txIQ) -> Product6/1
  FIR Interpolator/3 -> Terminator/1
  modEnable/1 -> Baseband Modulator/4(modEnable)
  OFDMmodType/1 -> Baseband Modulator/2(OFDMmodType)
  modSel/1 -> Baseband Modulator/1(modSel)
  tuningWord/1 -> NCO/1
  SCmodType/1 -> Baseband Modulator/3(SCmodType)
  FIR Interpolator1/3 -> Terminator1/1

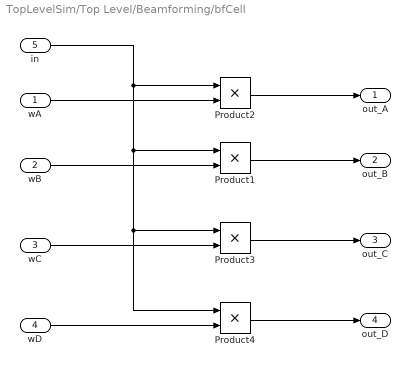
== system TopLevelSim/Top Level/Beamforming/bfCell ==
  wA : Inport
  wB : Inport  Port=2
  wC : Inport  Port=3
  wD : Inport  Port=4
  in : Inport  Port=5
  Product{1..4} (4 alike) : Product  OutDataTypeStr=fixdt(1,FXP.sampWL,FXP.sampFL)
  out_A : Outport
  out_B : Outport  Port=2
  out_C : Outport  Port=3
  out_D : Outport  Port=4
  wires:
  wB/1 -> Product1/2
  in/1 -> Product2/1, Product1/1, Product4/1, Product3/1
  wC/1 -> Product3/2
  wD/1 -> Product4/2
  Product3/1 -> out_C/1
  Product1/1 -> out_B/1
  Product4/1 -> out_D/1
  Product2/1 -> out_A/1
  wA/1 -> Product2/2

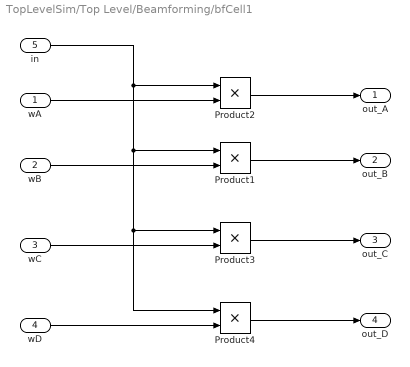
== system TopLevelSim/Top Level/Beamforming/bfCell1 ==
  wA : Inport
  wB : Inport  Port=2
  wC : Inport  Port=3
  wD : Inport  Port=4
  in : Inport  Port=5
  Product{1..4} (4 alike) : Product  OutDataTypeStr=fixdt(1,FXP.sampWL,FXP.sampFL)
  out_A : Outport
  out_B : Outport  Port=2
  out_C : Outport  Port=3
  out_D : Outport  Port=4
  wires:
  wA/1 -> Product2/2
  Product2/1 -> out_A/1
  Product4/1 -> out_D/1
  Product1/1 -> out_B/1
  Product3/1 -> out_C/1
  wD/1 -> Product4/2
  wC/1 -> Product3/2
  in/1 -> Product3/1, Product4/1, Product1/1, Product2/1
  wB/1 -> Product1/2

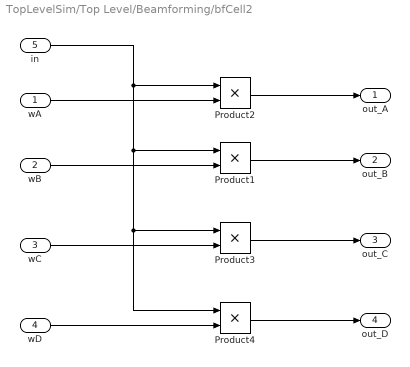
== system TopLevelSim/Top Level/Beamforming/bfCell2 ==
  wA : Inport
  wB : Inport  Port=2
  wC : Inport  Port=3
  wD : Inport  Port=4
  in : Inport  Port=5
  Product{1..4} (4 alike) : Product  OutDataTypeStr=fixdt(1,FXP.sampWL,FXP.sampFL)
  out_A : Outport
  out_B : Outport  Port=2
  out_C : Outport  Port=3
  out_D : Outport  Port=4
  wires:
  wB/1 -> Product1/2
  in/1 -> Product2/1, Product1/1, Product4/1, Product3/1
  wC/1 -> Product3/2
  wD/1 -> Product4/2
  Product3/1 -> out_C/1
  Product1/1 -> out_B/1
  Product4/1 -> out_D/1
  Product2/1 -> out_A/1
  wA/1 -> Product2/2

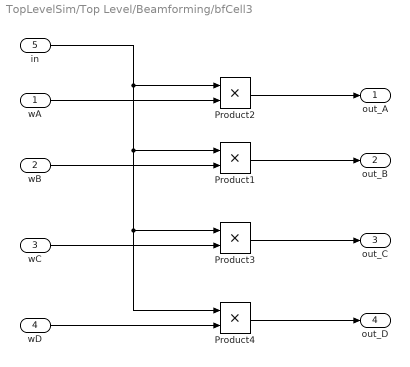
== system TopLevelSim/Top Level/Beamforming/bfCell3 ==
  wA : Inport
  wB : Inport  Port=2
  wC : Inport  Port=3
  wD : Inport  Port=4
  in : Inport  Port=5
  Product{1..4} (4 alike) : Product  OutDataTypeStr=fixdt(1,FXP.sampWL,FXP.sampFL)
  out_A : Outport
  out_B : Outport  Port=2
  out_C : Outport  Port=3
  out_D : Outport  Port=4
  wires:
  wA/1 -> Product2/2
  Product2/1 -> out_A/1
  Product4/1 -> out_D/1
  Product1/1 -> out_B/1
  Product3/1 -> out_C/1
  wD/1 -> Product4/2
  wC/1 -> Product3/2
  in/1 -> Product3/1, Product4/1, Product1/1, Product2/1
  wB/1 -> Product1/2

== system TopLevelSim/Top Level/Baseband Signal Generator/channel1/Baseband Modulator ==
  modSel : Inport
  OFDMmodType : Inport  Port=2
  SCmodType : Inport  Port=3
  modEnable : Inport  Port=4
  Constant2 : Constant  Value=complex(1,0)  OutDataTypeStr=fixdt(1,FXP.sampWL,FXP.sampFL)  SampleTime=sysParams.FPGAClkPeriod
  Counter Free-Running : hdlsllib/Sources/Counter Free-Running  NumBits=lutAddrWidth  tsamp=sysParams.FPGAClkPeriod
  Direct Lookup Table (n-D) : LookupNDDirect  NumberOfTableDimensions=1  Table=txData(:,1)  DiagnosticForOutOfRangeInput=Error
  OFDM Modulator : Subsystem
  SC Modulator : Subsystem
  Switch : Switch  Criteria=u2 > Threshold  OutDataTypeStr=fixdt(1,FXP.sampWL,FXP.sampFL)  SaturateOnIntegerOverflow=off  InputSameDT=off
  Switch1 : Switch  Criteria=u2 > Threshold  OutDataTypeStr=fixdt(1,FXP.sampWL,FXP.sampFL)  SaturateOnIntegerOverflow=off  InputSameDT=off
  txIQ : Outport
  wires:
  OFDMmodType/1 -> OFDM Modulator/2(OFDMmodType)
  Counter Free-Running/1 -> Direct Lookup Table (n-D)/1
  OFDM Modulator/1(txIQ) -> Switch1/3
  Direct Lookup Table (n-D)/1 -> SC Modulator/2(txBits), OFDM Modulator/1(txBits)
  SC Modulator/1(txIQ) -> Switch1/1
  SCmodType/1 -> SC Modulator/1(SCmodType)
  modSel/1 -> Switch1/2
  modEnable/1 -> Switch/2
  Switch1/1 -> Switch/1
  Switch/1 -> txIQ/1
  Constant2/1 -> Switch/3

== system TopLevelSim/Top Level/Baseband Signal Generator/channel2/Baseband Modulator ==
  modSel : Inport
  OFDMmodType : Inport  Port=2
  SCmodType : Inport  Port=3
  modEnable : Inport  Port=4
  Constant2 : Constant  Value=complex(1,0)  OutDataTypeStr=fixdt(1,FXP.sampWL,FXP.sampFL)  SampleTime=sysParams.FPGAClkPeriod
  Counter Free-Running : hdlsllib/Sources/Counter Free-Running  NumBits=lutAddrWidth  tsamp=sysParams.FPGAClkPeriod
  Direct Lookup Table (n-D) : LookupNDDirect  NumberOfTableDimensions=1  Table=txData(:,2)  DiagnosticForOutOfRangeInput=Error
  OFDM Modulator : Subsystem
  SC Modulator : Subsystem
  Switch : Switch  Criteria=u2 > Threshold  OutDataTypeStr=fixdt(1,FXP.sampWL,FXP.sampFL)  SaturateOnIntegerOverflow=off  InputSameDT=off
  Switch1 : Switch  Criteria=u2 > Threshold  OutDataTypeStr=fixdt(1,FXP.sampWL,FXP.sampFL)  SaturateOnIntegerOverflow=off  InputSameDT=off
  txIQ : Outport
  wires:
  Constant2/1 -> Switch/3
  Switch/1 -> txIQ/1
  Switch1/1 -> Switch/1
  modEnable/1 -> Switch/2
  modSel/1 -> Switch1/2
  SCmodType/1 -> SC Modulator/1(SCmodType)
  SC Modulator/1(txIQ) -> Switch1/1
  Direct Lookup Table (n-D)/1 -> OFDM Modulator/1(txBits), SC Modulator/2(txBits)
  OFDM Modulator/1(txIQ) -> Switch1/3
  Counter Free-Running/1 -> Direct Lookup Table (n-D)/1
  OFDMmodType/1 -> OFDM Modulator/2(OFDMmodType)

== system TopLevelSim/Top Level/Baseband Signal Generator/channel3/Baseband Modulator ==
  modSel : Inport
  OFDMmodType : Inport  Port=2
  SCmodType : Inport  Port=3
  modEnable : Inport  Port=4
  Constant2 : Constant  Value=complex(1,0)  OutDataTypeStr=fixdt(1,FXP.sampWL,FXP.sampFL)  SampleTime=sysParams.FPGAClkPeriod
  Counter Free-Running : hdlsllib/Sources/Counter Free-Running  NumBits=lutAddrWidth  tsamp=sysParams.FPGAClkPeriod
  Direct Lookup Table (n-D) : LookupNDDirect  NumberOfTableDimensions=1  Table=txData(:,3)  DiagnosticForOutOfRangeInput=Error
  OFDM Modulator : Subsystem
  SC Modulator : Subsystem
  Switch : Switch  Criteria=u2 > Threshold  OutDataTypeStr=fixdt(1,FXP.sampWL,FXP.sampFL)  SaturateOnIntegerOverflow=off  InputSameDT=off
  Switch1 : Switch  Criteria=u2 > Threshold  OutDataTypeStr=fixdt(1,FXP.sampWL,FXP.sampFL)  SaturateOnIntegerOverflow=off  InputSameDT=off
  txIQ : Outport
  wires:
  OFDMmodType/1 -> OFDM Modulator/2(OFDMmodType)
  Counter Free-Running/1 -> Direct Lookup Table (n-D)/1
  OFDM Modulator/1(txIQ) -> Switch1/3
  Direct Lookup Table (n-D)/1 -> SC Modulator/2(txBits), OFDM Modulator/1(txBits)
  SC Modulator/1(txIQ) -> Switch1/1
  SCmodType/1 -> SC Modulator/1(SCmodType)
  modSel/1 -> Switch1/2
  modEnable/1 -> Switch/2
  Switch1/1 -> Switch/1
  Switch/1 -> txIQ/1
  Constant2/1 -> Switch/3

== system TopLevelSim/Top Level/Baseband Signal Generator/channel4/Baseband Modulator ==
  modSel : Inport
  OFDMmodType : Inport  Port=2
  SCmodType : Inport  Port=3
  modEnable : Inport  Port=4
  Constant2 : Constant  Value=complex(1,0)  OutDataTypeStr=fixdt(1,FXP.sampWL,FXP.sampFL)  SampleTime=sysParams.FPGAClkPeriod
  Counter Free-Running : hdlsllib/Sources/Counter Free-Running  NumBits=lutAddrWidth  tsamp=sysParams.FPGAClkPeriod
  Direct Lookup Table (n-D) : LookupNDDirect  NumberOfTableDimensions=1  Table=txData(:,4)  DiagnosticForOutOfRangeInput=Error
  OFDM Modulator : Subsystem
  SC Modulator : Subsystem
  Switch : Switch  Criteria=u2 > Threshold  OutDataTypeStr=fixdt(1,FXP.sampWL,FXP.sampFL)  SaturateOnIntegerOverflow=off  InputSameDT=off
  Switch1 : Switch  Criteria=u2 > Threshold  OutDataTypeStr=fixdt(1,FXP.sampWL,FXP.sampFL)  SaturateOnIntegerOverflow=off  InputSameDT=off
  txIQ : Outport
  wires:
  Constant2/1 -> Switch/3
  Switch/1 -> txIQ/1
  Switch1/1 -> Switch/1
  modEnable/1 -> Switch/2
  modSel/1 -> Switch1/2
  SCmodType/1 -> SC Modulator/1(SCmodType)
  SC Modulator/1(txIQ) -> Switch1/1
  Direct Lookup Table (n-D)/1 -> OFDM Modulator/1(txBits), SC Modulator/2(txBits)
  OFDM Modulator/1(txIQ) -> Switch1/3
  Counter Free-Running/1 -> Direct Lookup Table (n-D)/1
  OFDMmodType/1 -> OFDM Modulator/2(OFDMmodType)

== system TopLevelSim/Top Level/Baseband Signal Generator/channel1/Baseband Modulator/OFDM Modulator ==
  txBits : Inport
  OFDMmodType : Inport  Port=2
  Constant : Constant  OutDataTypeStr=boolean  SampleTime=sysParams.FPGAClkPeriod
  OFDM Modulator : whdlmod/OFDM Modulator  OFDMParametersSource=Property  FFTLength=OFDM.ifftSize  MaxFFTLength=64  CPLength=OFDM.CpLength  numLgSc=OFDM.numLgSc  numRgSc=OFDM.numRgSc  InsertDCNull=off  Windowing=on  WindowLength=OFDM.WindowLength  MaxWindowLength=8  ResetInputPort=off  Normalize=on  RoundingMethod=Floor  SimulateUsing=Code generation
  Terminator : Terminator
  Terminator1 : Terminator
  mapper : Subsystem
  txIQ : Outport
  wires:
  txBits/1 -> mapper/1(txBits)
  OFDMmodType/1 -> mapper/2(OFDMmodType)
  OFDM Modulator/1 -> txIQ/1
  OFDM Modulator/2 -> Terminator1/1
  mapper/1(tx_IQ) -> OFDM Modulator/1
  OFDM Modulator/3 -> Terminator/1
  Constant/1 -> OFDM Modulator/2

== system TopLevelSim/Top Level/Baseband Signal Generator/channel1/Baseband Modulator/SC Modulator ==
  SCmodType : Inport
  txBits : Inport  Port=2
  FIR Interpolation : dspmlti4/FIR Interpolation  FilterSource=Dialog parameters  PrivateCoeffs=0  h=SC.firTaps  L=SC.firInterpFactor  FilterObject=FINTERP  framing=Allow multirate processing  outputBufInitCond=0  roundingMode=Floor  overflowMode=off  firstCoeffMode=Binary point scaling  firstCoeffWordLength=FXP.coeffWL  firstCoeffFracLength=FXP.coeffFL  firstCoeffDataTypeStr=fixdt(1,FXP.coeffWL,FXP.coeffFL)  firstCoeffMin=[]  firstCoeffMax=[]  firstCoeffLastDataTypeStr=fixdt(1,FXP.coeffWL,FXP.coeffFL)  outputMode=Binary point scaling  outputWordLength=FXP.sampWL  outputFracLength=FXP.sampFL  outputDataTypeStr=fixdt(1,FXP.sampWL,FXP.sampFL)  outputMin=[]  outputMax=[]  outputLastDataTypeStr=fixdt(1,FXP.sampWL,FXP.sampFL)
  Rate Transition : RateTransition  OutPortSampleTimeMultiple=40  OutPortSampleTime=1/SC.symRate
  Root-Raised Cosine : dspmlti4/FIR Interpolation  FilterSource=Dialog parameters  PrivateCoeffs=0  h=SC.RRC.taps  L=SC.RRC.sampPerSym  FilterObject=FINTERP  framing=Allow multirate processing  outputBufInitCond=0  roundingMode=Floor  overflowMode=off  firstCoeffMode=Binary point scaling  firstCoeffWordLength=FXP.coeffWL  firstCoeffFracLength=FXP.coeffFL  firstCoeffDataTypeStr=fixdt(1,FXP.coeffWL,FXP.coeffFL)  firstCoeffMin=[]  firstCoeffMax=[]  firstCoeffLastDataTypeStr=fixdt(1,FXP.coeffWL,FXP.coeffFL)  outputMode=Binary point scaling  outputWordLength=FXP.sampWL  outputFracLength=FXP.sampFL  outputDataTypeStr=fixdt(1,FXP.sampWL,FXP.sampFL)  outputMin=[]  outputMax=[]  outputLastDataTypeStr=fixdt(1,FXP.sampWL,FXP.sampFL)
  mapper : Subsystem
  txIQ : Outport
  wires:
  txBits/1 -> mapper/1(txBits)
  SCmodType/1 -> mapper/2(SCmodType)
  mapper/1(tx_IQ) -> Rate Transition/1
  Rate Transition/1 -> Root-Raised Cosine/1
  Root-Raised Cosine/1 -> FIR Interpolation/1
  FIR Interpolation/1 -> txIQ/1

== system TopLevelSim/Top Level/Baseband Signal Generator/channel2/Baseband Modulator/OFDM Modulator ==
  txBits : Inport
  OFDMmodType : Inport  Port=2
  Constant : Constant  OutDataTypeStr=boolean  SampleTime=sysParams.FPGAClkPeriod
  OFDM Modulator : whdlmod/OFDM Modulator  OFDMParametersSource=Property  FFTLength=OFDM.ifftSize  MaxFFTLength=64  CPLength=OFDM.CpLength  numLgSc=OFDM.numLgSc  numRgSc=OFDM.numRgSc  InsertDCNull=off  Windowing=on  WindowLength=OFDM.WindowLength  MaxWindowLength=8  ResetInputPort=off  Normalize=on  RoundingMethod=Floor  SimulateUsing=Code generation
  Terminator : Terminator
  Terminator1 : Terminator
  mapper : Subsystem
  txIQ : Outport
  wires:
  Constant/1 -> OFDM Modulator/2
  OFDM Modulator/3 -> Terminator/1
  mapper/1(tx_IQ) -> OFDM Modulator/1
  OFDM Modulator/2 -> Terminator1/1
  OFDM Modulator/1 -> txIQ/1
  OFDMmodType/1 -> mapper/2(OFDMmodType)
  txBits/1 -> mapper/1(txBits)

== system TopLevelSim/Top Level/Baseband Signal Generator/channel2/Baseband Modulator/SC Modulator ==
  SCmodType : Inport
  txBits : Inport  Port=2
  FIR Interpolation : dspmlti4/FIR Interpolation  FilterSource=Dialog parameters  PrivateCoeffs=0  h=SC.firTaps  L=SC.firInterpFactor  FilterObject=FINTERP  framing=Allow multirate processing  outputBufInitCond=0  roundingMode=Floor  overflowMode=off  firstCoeffMode=Binary point scaling  firstCoeffWordLength=FXP.coeffWL  firstCoeffFracLength=FXP.coeffFL  firstCoeffDataTypeStr=fixdt(1,FXP.coeffWL,FXP.coeffFL)  firstCoeffMin=[]  firstCoeffMax=[]  firstCoeffLastDataTypeStr=fixdt(1,FXP.coeffWL,FXP.coeffFL)  outputMode=Binary point scaling  outputWordLength=FXP.sampWL  outputFracLength=FXP.sampFL  outputDataTypeStr=fixdt(1,FXP.sampWL,FXP.sampFL)  outputMin=[]  outputMax=[]  outputLastDataTypeStr=fixdt(1,FXP.sampWL,FXP.sampFL)
  Rate Transition : RateTransition  OutPortSampleTimeMultiple=40  OutPortSampleTime=1/SC.symRate
  Root-Raised Cosine : dspmlti4/FIR Interpolation  FilterSource=Dialog parameters  PrivateCoeffs=0  h=SC.RRC.taps  L=SC.RRC.sampPerSym  FilterObject=FINTERP  framing=Allow multirate processing  outputBufInitCond=0  roundingMode=Floor  overflowMode=off  firstCoeffMode=Binary point scaling  firstCoeffWordLength=FXP.coeffWL  firstCoeffFracLength=FXP.coeffFL  firstCoeffDataTypeStr=fixdt(1,FXP.coeffWL,FXP.coeffFL)  firstCoeffMin=[]  firstCoeffMax=[]  firstCoeffLastDataTypeStr=fixdt(1,FXP.coeffWL,FXP.coeffFL)  outputMode=Binary point scaling  outputWordLength=FXP.sampWL  outputFracLength=FXP.sampFL  outputDataTypeStr=fixdt(1,FXP.sampWL,FXP.sampFL)  outputMin=[]  outputMax=[]  outputLastDataTypeStr=fixdt(1,FXP.sampWL,FXP.sampFL)
  mapper : Subsystem
  txIQ : Outport
  wires:
  FIR Interpolation/1 -> txIQ/1
  Root-Raised Cosine/1 -> FIR Interpolation/1
  Rate Transition/1 -> Root-Raised Cosine/1
  mapper/1(tx_IQ) -> Rate Transition/1
  SCmodType/1 -> mapper/2(SCmodType)
  txBits/1 -> mapper/1(txBits)

== system TopLevelSim/Top Level/Baseband Signal Generator/channel3/Baseband Modulator/OFDM Modulator ==
  txBits : Inport
  OFDMmodType : Inport  Port=2
  Constant : Constant  OutDataTypeStr=boolean  SampleTime=sysParams.FPGAClkPeriod
  OFDM Modulator : whdlmod/OFDM Modulator  OFDMParametersSource=Property  FFTLength=OFDM.ifftSize  MaxFFTLength=64  CPLength=OFDM.CpLength  numLgSc=OFDM.numLgSc  numRgSc=OFDM.numRgSc  InsertDCNull=off  Windowing=on  WindowLength=OFDM.WindowLength  MaxWindowLength=8  ResetInputPort=off  Normalize=on  RoundingMethod=Floor  SimulateUsing=Code generation
  Terminator : Terminator
  Terminator1 : Terminator
  mapper : Subsystem
  txIQ : Outport
  wires:
  txBits/1 -> mapper/1(txBits)
  OFDMmodType/1 -> mapper/2(OFDMmodType)
  OFDM Modulator/1 -> txIQ/1
  OFDM Modulator/2 -> Terminator1/1
  mapper/1(tx_IQ) -> OFDM Modulator/1
  OFDM Modulator/3 -> Terminator/1
  Constant/1 -> OFDM Modulator/2

== system TopLevelSim/Top Level/Baseband Signal Generator/channel3/Baseband Modulator/SC Modulator ==
  SCmodType : Inport
  txBits : Inport  Port=2
  FIR Interpolation : dspmlti4/FIR Interpolation  FilterSource=Dialog parameters  PrivateCoeffs=0  h=SC.firTaps  L=SC.firInterpFactor  FilterObject=FINTERP  framing=Allow multirate processing  outputBufInitCond=0  roundingMode=Floor  overflowMode=off  firstCoeffMode=Binary point scaling  firstCoeffWordLength=FXP.coeffWL  firstCoeffFracLength=FXP.coeffFL  firstCoeffDataTypeStr=fixdt(1,FXP.coeffWL,FXP.coeffFL)  firstCoeffMin=[]  firstCoeffMax=[]  firstCoeffLastDataTypeStr=fixdt(1,FXP.coeffWL,FXP.coeffFL)  outputMode=Binary point scaling  outputWordLength=FXP.sampWL  outputFracLength=FXP.sampFL  outputDataTypeStr=fixdt(1,FXP.sampWL,FXP.sampFL)  outputMin=[]  outputMax=[]  outputLastDataTypeStr=fixdt(1,FXP.sampWL,FXP.sampFL)
  Rate Transition : RateTransition  OutPortSampleTimeMultiple=40  OutPortSampleTime=1/SC.symRate
  Root-Raised Cosine : dspmlti4/FIR Interpolation  FilterSource=Dialog parameters  PrivateCoeffs=0  h=SC.RRC.taps  L=SC.RRC.sampPerSym  FilterObject=FINTERP  framing=Allow multirate processing  outputBufInitCond=0  roundingMode=Floor  overflowMode=off  firstCoeffMode=Binary point scaling  firstCoeffWordLength=FXP.coeffWL  firstCoeffFracLength=FXP.coeffFL  firstCoeffDataTypeStr=fixdt(1,FXP.coeffWL,FXP.coeffFL)  firstCoeffMin=[]  firstCoeffMax=[]  firstCoeffLastDataTypeStr=fixdt(1,FXP.coeffWL,FXP.coeffFL)  outputMode=Binary point scaling  outputWordLength=FXP.sampWL  outputFracLength=FXP.sampFL  outputDataTypeStr=fixdt(1,FXP.sampWL,FXP.sampFL)  outputMin=[]  outputMax=[]  outputLastDataTypeStr=fixdt(1,FXP.sampWL,FXP.sampFL)
  mapper : Subsystem
  txIQ : Outport
  wires:
  txBits/1 -> mapper/1(txBits)
  SCmodType/1 -> mapper/2(SCmodType)
  mapper/1(tx_IQ) -> Rate Transition/1
  Rate Transition/1 -> Root-Raised Cosine/1
  Root-Raised Cosine/1 -> FIR Interpolation/1
  FIR Interpolation/1 -> txIQ/1

== system TopLevelSim/Top Level/Baseband Signal Generator/channel4/Baseband Modulator/OFDM Modulator ==
  txBits : Inport
  OFDMmodType : Inport  Port=2
  Constant : Constant  OutDataTypeStr=boolean  SampleTime=sysParams.FPGAClkPeriod
  OFDM Modulator : whdlmod/OFDM Modulator  OFDMParametersSource=Property  FFTLength=OFDM.ifftSize  MaxFFTLength=64  CPLength=OFDM.CpLength  numLgSc=OFDM.numLgSc  numRgSc=OFDM.numRgSc  InsertDCNull=off  Windowing=on  WindowLength=OFDM.WindowLength  MaxWindowLength=8  ResetInputPort=off  Normalize=on  RoundingMethod=Floor  SimulateUsing=Code generation
  Terminator : Terminator
  Terminator1 : Terminator
  mapper : Subsystem
  txIQ : Outport
  wires:
  Constant/1 -> OFDM Modulator/2
  OFDM Modulator/3 -> Terminator/1
  mapper/1(tx_IQ) -> OFDM Modulator/1
  OFDM Modulator/2 -> Terminator1/1
  OFDM Modulator/1 -> txIQ/1
  OFDMmodType/1 -> mapper/2(OFDMmodType)
  txBits/1 -> mapper/1(txBits)

== system TopLevelSim/Top Level/Baseband Signal Generator/channel4/Baseband Modulator/SC Modulator ==
  SCmodType : Inport
  txBits : Inport  Port=2
  FIR Interpolation : dspmlti4/FIR Interpolation  FilterSource=Dialog parameters  PrivateCoeffs=0  h=SC.firTaps  L=SC.firInterpFactor  FilterObject=FINTERP  framing=Allow multirate processing  outputBufInitCond=0  roundingMode=Floor  overflowMode=off  firstCoeffMode=Binary point scaling  firstCoeffWordLength=FXP.coeffWL  firstCoeffFracLength=FXP.coeffFL  firstCoeffDataTypeStr=fixdt(1,FXP.coeffWL,FXP.coeffFL)  firstCoeffMin=[]  firstCoeffMax=[]  firstCoeffLastDataTypeStr=fixdt(1,FXP.coeffWL,FXP.coeffFL)  outputMode=Binary point scaling  outputWordLength=FXP.sampWL  outputFracLength=FXP.sampFL  outputDataTypeStr=fixdt(1,FXP.sampWL,FXP.sampFL)  outputMin=[]  outputMax=[]  outputLastDataTypeStr=fixdt(1,FXP.sampWL,FXP.sampFL)
  Rate Transition : RateTransition  OutPortSampleTimeMultiple=40  OutPortSampleTime=1/SC.symRate
  Root-Raised Cosine : dspmlti4/FIR Interpolation  FilterSource=Dialog parameters  PrivateCoeffs=0  h=SC.RRC.taps  L=SC.RRC.sampPerSym  FilterObject=FINTERP  framing=Allow multirate processing  outputBufInitCond=0  roundingMode=Floor  overflowMode=off  firstCoeffMode=Binary point scaling  firstCoeffWordLength=FXP.coeffWL  firstCoeffFracLength=FXP.coeffFL  firstCoeffDataTypeStr=fixdt(1,FXP.coeffWL,FXP.coeffFL)  firstCoeffMin=[]  firstCoeffMax=[]  firstCoeffLastDataTypeStr=fixdt(1,FXP.coeffWL,FXP.coeffFL)  outputMode=Binary point scaling  outputWordLength=FXP.sampWL  outputFracLength=FXP.sampFL  outputDataTypeStr=fixdt(1,FXP.sampWL,FXP.sampFL)  outputMin=[]  outputMax=[]  outputLastDataTypeStr=fixdt(1,FXP.sampWL,FXP.sampFL)
  mapper : Subsystem
  txIQ : Outport
  wires:
  FIR Interpolation/1 -> txIQ/1
  Root-Raised Cosine/1 -> FIR Interpolation/1
  Rate Transition/1 -> Root-Raised Cosine/1
  mapper/1(tx_IQ) -> Rate Transition/1
  SCmodType/1 -> mapper/2(SCmodType)
  txBits/1 -> mapper/1(txBits)
